simulink model "differential_flatness"  (R2015a)
settings: Solver=ode45  StartTime=0.0  StopTime=inf  FixedStep=0.001  RelTol=1e-3
values from neighbouring files (symbols this model uses):
  colors = [colors;colors_rotor]    [sketch_copter.m]
  F = thrust_c    [attitude_controller.m]    (also in quad_dynamics.m = uu(1); sketch_copter.m = [F;F_rotor+rotor*size(V_rotor,1)]; testing_dynamics.m = uu(1))
  forces_moments = [fz; l; m; n]    [forces_moments.m]
  V = V*R    [drawAircraft.m]    (also in sketch_copter.m = [V;V_rotor*R]; testing_drawAircraft.m)
undefined symbols (not defined in the file or in its folder): attitude_controller, diff_flat, drawAircraft, inverse, lqr_controller, P, trajectory
settings Model: NumberOfSteps=100  Creator=ecestudent  LastModifiedBy=ecestudent

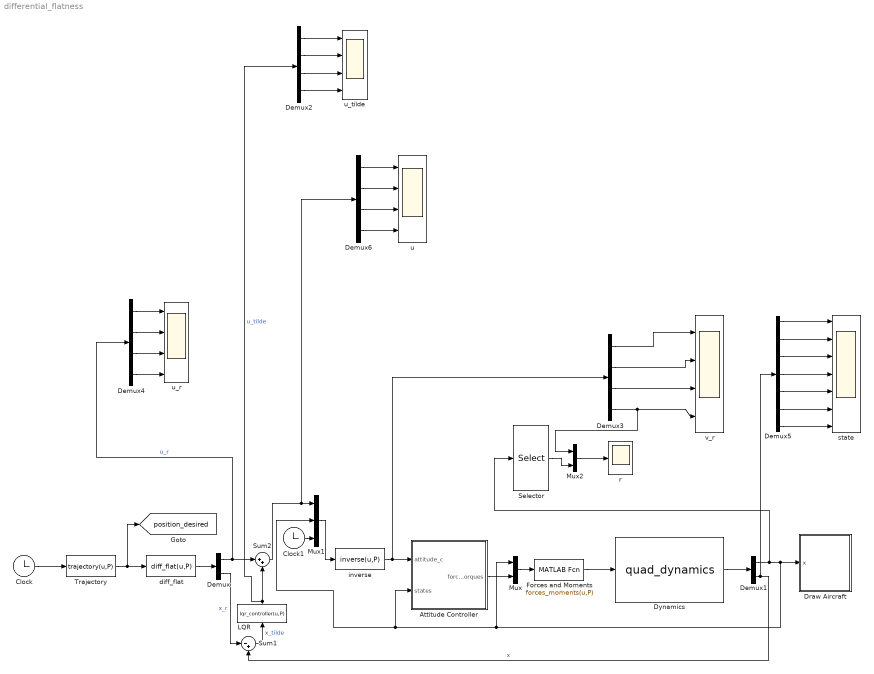
== system differential_flatness ==
  Attitude Controller : Subsystem
      mask Display: image(imread('images/auto_pilot.jpg'))
  Clock : Clock
  Clock1 : Clock
  Demux : Demux  Outputs=[4 7]
  Demux1 : Demux  Outputs=[12 7]
  Demux{2..4,6} (4 alike) : Demux
  Demux5 : Demux  Outputs=7
  Draw Aircraft : Subsystem
      mask Display: image(imread('images/tv.jpg'))
  Dynamics : S-Function  FunctionName=quad_dynamics  Parameters=P
      mask Display: image(imread('images/hexacopter.png'))
  Forces and Moments : MATLABFcn  MATLABFcn=forces_moments(u,P)  OutputDimensions=4
  LQR : MATLABFcn  MATLABFcn=lqr_controller(u,P)  OutputDimensions=4
  Mux : Mux  Inputs=2
  Mux1 : Mux  Inputs=3
  Mux2 : Mux  Inputs=2
  Selector : Selector  InputPortWidth=12  Indices=[12]
  Sum1 : Sum  Inputs=|-+
  Sum2 : Sum  Inputs=|++
  Trajectory : MATLABFcn  MATLABFcn=trajectory(u,P)  OutputDimensions=11
  diff_flat : MATLABFcn  MATLABFcn=diff_flat(u,P)  OutputDimensions=11
  inverse : MATLABFcn  MATLABFcn=inverse(u,P)  OutputDimensions=4
  r : Scope
      settings: TimeRange=1.839020215818323  YMin=-4.25e-26  YMax=5e-27  SaveName=ScopeData3
  state : Scope  NumInputPorts=7
      settings: TimeRange=9.998000000000001  YMin=-1~-1~0~-1~-1~-0.5~-1  YMax=1~1~3~1~1~0.5~1  SaveName=ScopeData2
  u : Scope  NumInputPorts=4
      settings: YMin=-1~-6.775e-15~9.853~4.9375e-16  YMax=1~-6.625e-15~9.862~4.9625e-16  SaveName=ScopeData6
  u_r : Scope  NumInputPorts=4
      settings: YMin=-1~-1~-9.81~-1  YMax=1~1~-9.81~1
  u_tilde : Scope  NumInputPorts=4
      settings: YMin=-1~4e-22~2e-08~-3.5e-23  YMax=1~1.5e-21~1.1e-07~-7.5e-24  SaveName=ScopeData4
  v_r : Scope  NumInputPorts=4
      settings: TimeRange=1.839020215818323  YMin=37.3725~-3.5e-13~-1~-1  YMax=37.373~2.5e-13~1~1
  tag scope: position_desired=global
  wires:
  Clock/1 -> Trajectory/1
  Trajectory/1 -> [position_desired], diff_flat/1
  Mux/1 -> Forces and Moments/1
  Attitude Controller/1(force_torques) -> Mux/2
  Forces and Moments/1 -> Dynamics/1
  diff_flat/1 -> Demux/1
  Demux/1 -> Demux4/1, Sum2/1  "u_r"
  Demux/2 -> Sum1/1  "x_r"
  Dynamics/1 -> Demux1/1
  Demux1/1 -> Selector/1, Draw Aircraft/1(x), Attitude Controller/2(states), Mux1/2, Mux/1
  Demux1/2 -> Demux5/1, Sum1/2  "x"
  Sum1/1 -> LQR/1  "x_tilde"
  LQR/1 -> Sum2/2, Demux2/1  "u_tilde"
  Sum2/1 -> Demux6/1, Mux1/1
  Mux1/1 -> inverse/1
  Clock1/1 -> Mux1/3
  Demux2/1 -> u_tilde/1
  Demux2/2 -> u_tilde/2
  Demux2/3 -> u_tilde/3
  Demux2/4 -> u_tilde/4
  inverse/1 -> Attitude Controller/1(attitude_c), Demux3/1
  Demux3/1 -> v_r/1
  Demux3/2 -> v_r/2
  Demux3/3 -> v_r/3
  Demux3/4 -> Mux2/1, v_r/4
  Demux4/1 -> u_r/1
  Demux4/2 -> u_r/2
  Demux4/3 -> u_r/3
  Demux4/4 -> u_r/4
  Demux5/1 -> state/1
  Demux5/2 -> state/2
  Demux5/3 -> state/3
  Demux5/4 -> state/4
  Demux5/5 -> state/5
  Demux5/6 -> state/6
  Demux5/7 -> state/7
  Selector/1 -> Mux2/2
  Mux2/1 -> r/1
  Demux6/1 -> u/1
  Demux6/2 -> u/2
  Demux6/3 -> u/3
  Demux6/4 -> u/4

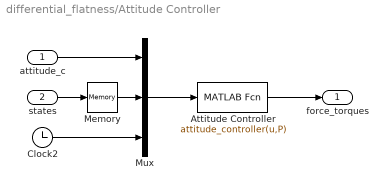
== system differential_flatness/Attitude Controller ==
  attitude_c : Inport
  states : Inport  Port=2
  Attitude Controller : MATLABFcn  MATLABFcn=attitude_controller(u,P)  OutputDimensions=4  SampleTime=0.002
  Clock2 : Clock
  Memory : Memory
  Mux : Mux  Inputs=3
  force_torques : Outport
  wires:
  Clock2/1 -> Mux/3
  Mux/1 -> Attitude Controller/1
  Attitude Controller/1 -> force_torques/1
  states/1 -> Memory/1
  attitude_c/1 -> Mux/1
  Memory/1 -> Mux/2

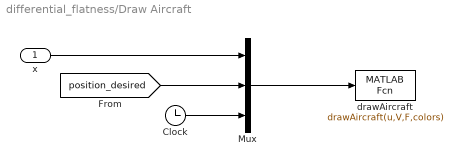
== system differential_flatness/Draw Aircraft ==
  x : Inport
  Clock : Clock
  Mux : Mux  Inputs=3
  drawAircraft : MATLABFcn  MATLABFcn=drawAircraft(u,V,F,colors)  OutputDimensions=0  SampleTime=0.1
  wires:
  x/1 -> Mux/1
  [position_desired] -> Mux/2
  Mux/1 -> drawAircraft/1
  Clock/1 -> Mux/3
